simulink model "PID_IMC_SL"  (R2023b)
settings: Solver=VariableStepAuto  StartTime=0.0  StopTime=30  RelTol=1e-3
libraries: cstblocks x2
settings Model: Creator=marif  LastModifiedBy=marif

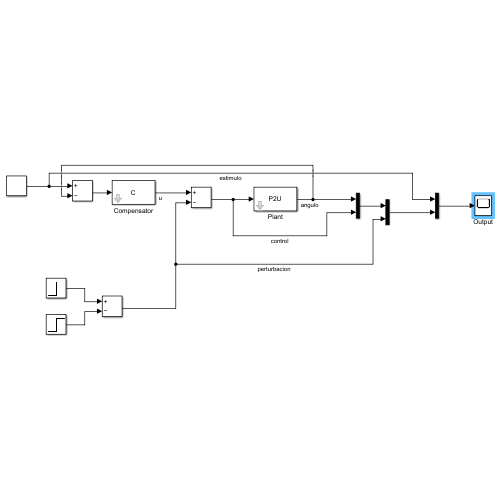
[thumbnail: Simulink's stored preview of the top-level diagram]
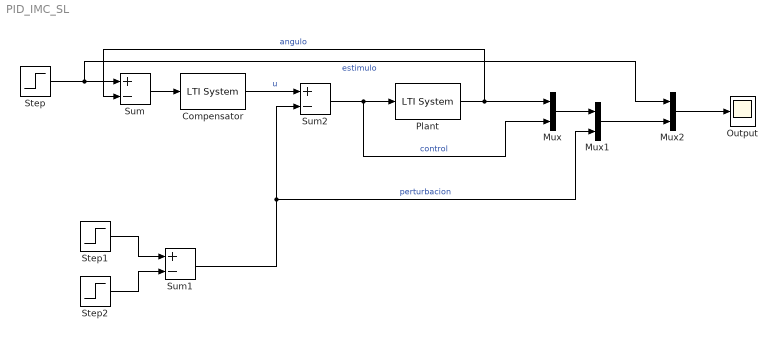
== system PID_IMC_SL ==
  Compensator : cstblocks/LTI System  sys=C  IC=[]  PadeOrder=0
  Mux : Mux  Inputs=2
  Mux1 : Mux  Inputs=2
  Mux2 : Mux  Inputs=2
  Output : Scope
  Plant : cstblocks/LTI System  sys=P2U  IC=[]  PadeOrder=0
  Step : Step  After=0.6  SampleTime=0
  Step1 : Step  Time=12  After=0.1  SampleTime=0
  Step2 : Step  Time=13  After=0.1  SampleTime=0
  Sum : Sum  Inputs=+-
  Sum1 : Sum  Inputs=+-
  Sum2 : Sum  Inputs=+-
  wires:
  Sum/1 -> Compensator/1
  Plant/1 -> Sum/2, Mux/1  "angulo"
  Step/1 -> Mux2/1, Sum/1  "estimulo"
  Sum2/1 -> Mux/2, Plant/1  "control"
  Compensator/1 -> Sum2/1  "u"
  Sum1/1 -> Mux1/2, Sum2/2  "perturbacion"
  Step1/1 -> Sum1/1
  Step2/1 -> Sum1/2
  Mux/1 -> Mux1/1
  Mux1/1 -> Mux2/2
  Mux2/1 -> Output/1
